simulink model "ZweiServer_EineWarteschlange"  (R2016a)
settings: Solver=VariableStepAuto  StartTime=0.0  StopTime=6000  RelTol=1e-3
undefined symbols (not defined in the file): elapsedTime, entity, m
settings Model: Creator=gome  LastModifiedBy=gome

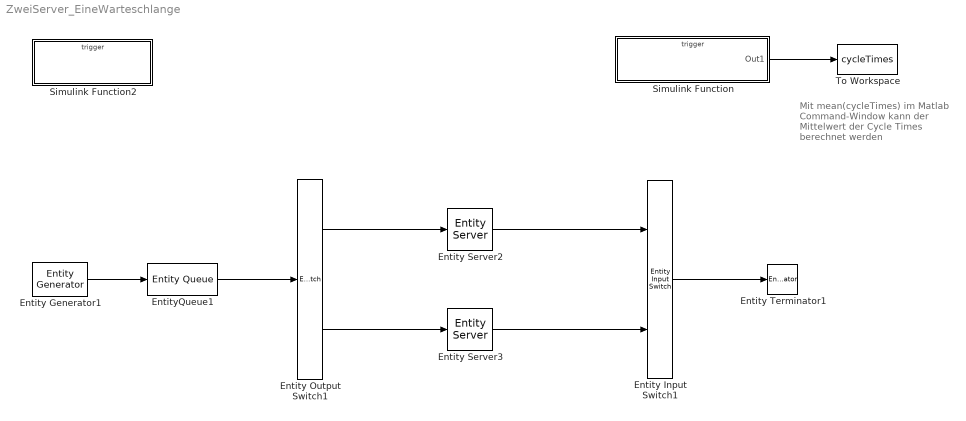
== system ZweiServer_EineWarteschlange ==
  note: Mit mean(cycleTimes) im Matlab Command-Window kann der Mittelwert der Cycle Times berechnet werden
  Entity Input Switch1 : EntityInputSwitch  InputPortMessageModes=m,m  OutputPortMessageModes=m
  Entity Output Switch1 : EntityOutputSwitch  InputPortMessageModes=m  OutputPortMessageModes=m,m  SwitchAttributeName=portNumber
  Entity Generator1 : EntityGenerator  OutputPortMessageModes=m  TimeSource=MATLAB action  IntergenerationTimeAction=dt = exprnd(0.5);  GenerateAction=entity.TimeStamp = stampEntity();  AttributeName=TimeStamp  EntityType=Structured  EntityTypeName=Entity
  Entity Server2 : EntityServer  InputPortMessageModes=m  OutputPortMessageModes=m  Capacity=1  ServiceTimeSource=MATLAB action  ServiceTimeAction=dt = exprnd(0.6);
  Entity Server3 : EntityServer  InputPortMessageModes=m  OutputPortMessageModes=m  Capacity=1  ServiceTimeSource=MATLAB action  ServiceTimeAction=dt = exprnd(0.6);
  Entity Terminator1 : EntityTerminator  InputPortMessageModes=m  EntryAction=elapsedTime(entity.TimeStamp);
  EntityQueue1 : EntityQueue  InputPortMessageModes=m  OutputPortMessageModes=m  Capacity=inf
      settings: OutputPortMap=o5
  Simulink Function : Subsystem  TreatAsAtomicUnit=on
  Simulink Function2 : Subsystem  TreatAsAtomicUnit=on
  To Workspace : ToWorkspace  VariableName=cycleTimes  SampleTime=-1
      settings: InputPortMessageModes=m
  wires:
  Simulink Function/1(Out1) -> To Workspace/1
  Entity Output Switch1/2 -> Entity Server3/1
  Entity Server2/1 -> Entity Input Switch1/1
  Entity Server3/1 -> Entity Input Switch1/2
  Entity Input Switch1/1 -> Entity Terminator1/1
  Entity Generator1/1 -> EntityQueue1/1
  EntityQueue1/1 -> Entity Output Switch1/1
  Entity Output Switch1/1 -> Entity Server2/1

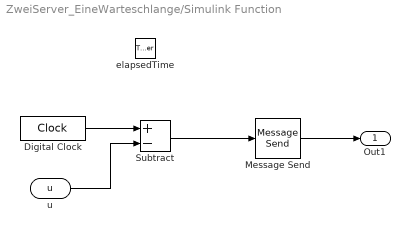
== system ZweiServer_EineWarteschlange/Simulink Function ==
  elapsedTime : TriggerPort  TriggerType=function-call  IsSimulinkFunction=on  FunctionName=elapsedTime  VariantControl=Variant
  Digital Clock : DigitalClock  SampleTime=-1
  Message Send : MessageSend  OutputPortMessageModes=m
      settings: InputPortMap=u1
  Subtract : Sum  Inputs=+-
  u : ArgIn  DisableCoverage=on  ArgumentName=u
  Out1 : Outport
  wires:
  Digital Clock/1 -> Subtract/1
  u/1 -> Subtract/2
  Subtract/1 -> Message Send/1
  Message Send/1 -> Out1/1

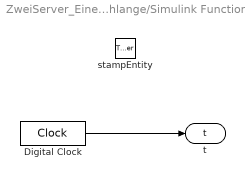
== system ZweiServer_EineWarteschlange/Simulink Function2 ==
  stampEntity : TriggerPort  TriggerType=function-call  IsSimulinkFunction=on  FunctionName=stampEntity  VariantControl=Variant
  Digital Clock : DigitalClock  SampleTime=-1
  t : ArgOut  DisableCoverage=on  ArgumentName=t
  wires:
  Digital Clock/1 -> t/1
